simulink model "modell2b"  (Simulink 6.1)
settings: Solver=ode3  StartTime=0.0  StopTime=15  FixedStep=0.02  RelTol=1e-3
settings Model: LastModifiedBy=Harkay T
settings DebuggingCC: SolverPrmCheckMsg=warning

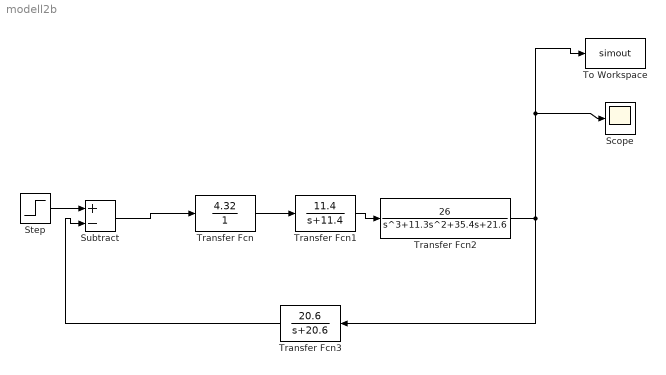
== system modell2b ==
  Scope : Scope
      settings: SaveName=SD  DataFormat=Array
  Step : Step  Time=0  SampleTime=0
  Subtract : Sum  Inputs=+-  OutScaling=2^-10
  To Workspace : ToWorkspace  VariableName=simout  SampleTime=-1  SaveFormat=Array
  Transfer Fcn : TransferFcn  Numerator=[4.32]  Denominator=[1 ]
  Transfer Fcn1 : TransferFcn  Numerator=[11.4]  Denominator=[1 11.4]
  Transfer Fcn2 : TransferFcn  Numerator=[26]  Denominator=[1 11.3 35.4 21.6]
  Transfer Fcn3 : TransferFcn  Orientation=left  Numerator=[20.6]  Denominator=[1 20.6]
  wires:
  Step/1 -> Subtract/1
  Subtract/1 -> Transfer Fcn/1
  Transfer Fcn/1 -> Transfer Fcn1/1
  Transfer Fcn1/1 -> Transfer Fcn2/1
  Transfer Fcn2/1 -> Transfer Fcn3/1, Scope/1, To Workspace/1
  Transfer Fcn3/1 -> Subtract/2
